simulink model "Tire2"  (R2017a)
settings: Solver=FixedStepAuto  StartTime=0.0  StopTime=10.0  FixedStep=.01  MaxStep=.01  RelTol=1e-3
libraries: simulink x2
settings Model: Creator=shant  LastModifiedBy=shant

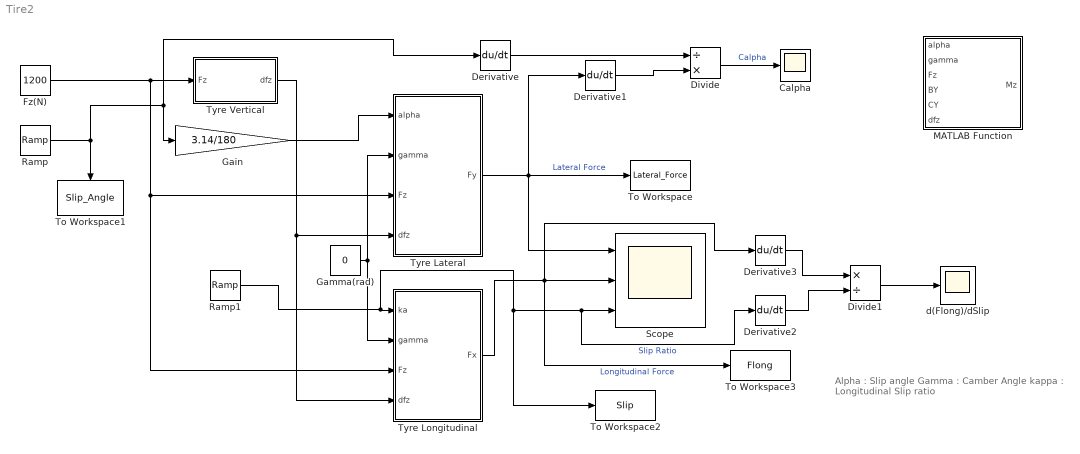
== system Tire2 ==
  note: Alpha : Slip angle
      | Gamma : Camber Angle
      | kappa : Longitudinal Slip ratio
  Calpha : Scope
  Derivative{,1..3} (4 alike) : Derivative
  Divide : Product  Inputs=/*
  Divide1 : Product  Inputs=*/
  Fz(N) : Constant  Value=1200
  Gain : Gain  Gain=3.14/180
  Gamma(rad) : Constant  Value=0
  MATLAB Function : MATLAB Function  TreatAsAtomicUnit=on
  Ramp : simulink/Sources/Ramp  slope=2  start=0  X0=-10
  Ramp1 : simulink/Sources/Ramp  slope=0  start=0  X0=0
  Scope : Scope  NumInputPorts=3
  To Workspace : ToWorkspace  VariableName=Lateral_Force  SampleTime=-1
  To Workspace1 : ToWorkspace  VariableName=Slip_Angle  SampleTime=-1
  To Workspace2 : ToWorkspace  VariableName=Slip  SampleTime=-1
  To Workspace3 : ToWorkspace  VariableName=Flong  SampleTime=-1
  Tyre Lateral : MATLAB Function  TreatAsAtomicUnit=on
  Tyre Longitudinal : MATLAB Function  TreatAsAtomicUnit=on
  Tyre Vertical : MATLAB Function  TreatAsAtomicUnit=on
  d(Flong)/dSlip : Scope
  wires:
  Fz(N)/1 -> Tyre Longitudinal/3(Fz), Tyre Lateral/3(Fz), Tyre Vertical/1(Fz)
  Tyre Vertical/1(dfz) -> Tyre Lateral/4(dfz), Tyre Longitudinal/4(dfz)
  Gamma(rad)/1 -> Tyre Lateral/2(gamma), Tyre Longitudinal/2(gamma)
  Ramp1/1 -> Tyre Longitudinal/1(ka), To Workspace2/1, Derivative2/1, Scope/3  "Slip Ratio"
  Tyre Lateral/1(Fy) -> Scope/1, To Workspace/1, Derivative1/1  "Lateral Force"
  Tyre Longitudinal/1(Fx) -> Derivative3/1, Scope/2, To Workspace3/1  "Longitudinal Force"
  Gain/1 -> Tyre Lateral/1(alpha)
  Ramp/1 -> Derivative/1, Gain/1, To Workspace1/1
  Divide/1 -> Calpha/1  "Calpha"
  Divide1/1 -> d(Flong)/dSlip/1
  Derivative2/1 -> Divide1/2
  Derivative3/1 -> Divide1/1
  Derivative1/1 -> Divide/2
  Derivative/1 -> Divide/1

== matlab function Tire2/Tyre Lateral ==
  data: alpha input; Fy output; gamma input; Fz input; dfz input
%function [Fy, BY, CY] = fcn(alpha, gamma, Fz, dfz)
function Fy  = fcn(alpha, gamma, Fz, dfz)
%a = evalin('ws', 'FtireS1');
gammaY = gamma;
Svy = Fz*((0 + 0*dfz)*1 + (-2.713 + -1.517*dfz)*gammaY)*1;
Shy = (0 + 0*dfz)*1 + -0.-203*gammaY;
alphaY = alpha + Shy;
Ey = (-0.4869 + -1.487*dfz)*(1- (0.06282 + 1.154*gammaY)*sign(alphaY))*1;
muY = (2.716 + -0.5444*dfz)*(1-5.19*(gammaY)^2)*1;
KY = -53.22*800*sin(2*atan(Fz/(2.06*800*1)))*(1-0.8336*abs(gammaY))*1*1;
DY = muY*Fz;
CY = 1.434*1;
BY = KY/(CY*DY);
Fy = DY*sin(CY*atan(BY*alphaY - Ey*(BY*alphaY-atan(BY*alphaY))))+Svy;

== matlab function Tire2/Tyre Vertical ==
  data: dfz output; Fz input
function dfz = fcn(Fz) %input Fzo, Ro, ka, alpha, gamma, Fz
%coder.extrinsic('evalin');
%a = evalin('ws', 'a');
Fzo  = 800; % Nominal vertical load
Fzoa = Fzo; % Load correction

dfz = (Fz - Fzoa)/Fzoa; % corrected Load
end

== matlab function Tire2/Tyre Longitudinal ==
  data: ka input; Fx output; gamma input; Fz input; dfz input
function Fx = fcn(ka, gamma, Fz, dfz)
%a = evalin('ws', 'FtireS1');
gammaX = gamma*1;
Shx = (0 + 0*dfz)*1;
kaX = ka + Shx;
Svx = Fz*(0 + 0*dfz)*1*1;
muX = (2.85 + -0.354*dfz)*(1 - 12.23*(gammaX)^2)*1;
Ex = (0.871 + -0.038*dfz + 0*(dfz)^2)*(1-0.071*sign(kaX))*1;
KX = Fz*(81.25 + -20.25*dfz)*exp(0.5*dfz)*1;
DX = muX*Fz;
CX = 1.786*1;
BX = KX/(CX*DX);
Fx = DX*sin(CX*atan(BX*kaX - Ex*(BX*kaX - atan(BX*kaX)))) + Svx;

== matlab function Tire2/MATLAB Function ==
  data: alpha input; Mz output; gamma input; Fz input; BY input; CY input; dfz input
function Mz = fcn(alpha, gamma, Fz, BY, CY, dfz)
gammaz = gamma*1;
Sht = (.208 + -.184*dfz)*gammaz;
Et = (-1.11 + -.265*dfz + -1.71*(dfz)^2);
Dr = Fz((-.00155 + -.0132*dfz) + (-1.09 + -.199*dfz)*gammaz)*.235;
Dt = Fz(.122 + -.0155*dfz)*(1 + -.0473*gammaz + -12.1*(gammaz)^2)*(.235/800)*1;
Bt = (11.8 + .16*dfz + -2.5*(dfz)^2)*(1 + 8.71*gammaz + 8.09*abs(gammaz));
Br = (-28.3 + -4*BY*CY);
Ct = 1.26;
alphat = alpha + Sht;
t = Dt*cos(Ct*atan(Bt*alphat - Et*(Bt*alphat - atan(Bt*alphat))))*cos(alpha);
